simulink model "up_counter_3bit"  (R2025b)
settings: Solver=VariableStepAuto  StartTime=0.0  StopTime=10.0  RelTol=1e-3
libraries: simulink_extras x4
settings Model: Creator=Johan  LastModifiedBy=Johan

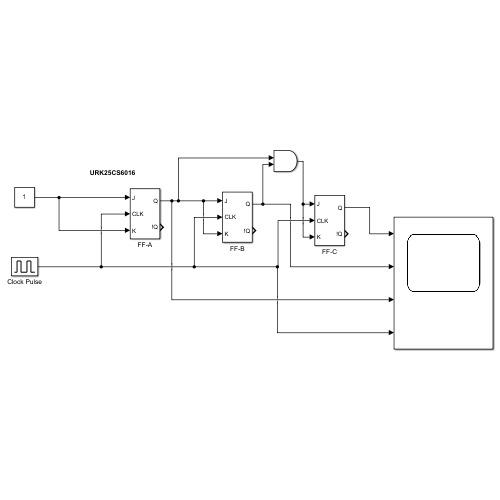
[thumbnail: Simulink's stored preview of the top-level diagram]
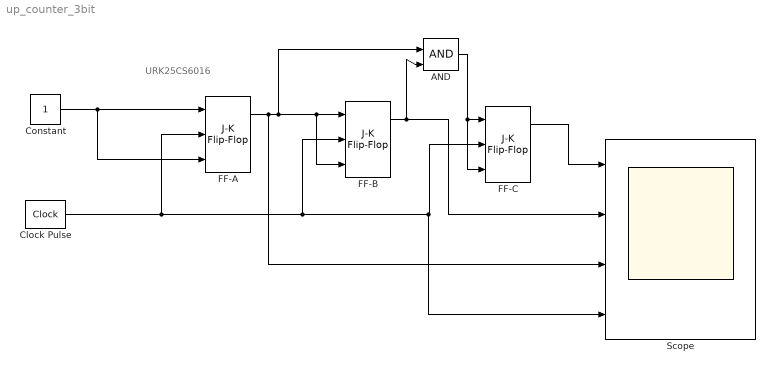
== system up_counter_3bit ==
  note: URK25CS6016
  AND : Logic  IconShape=distinctive  AllPortsSameDT=off  OutDataTypeStr=boolean
  Clock Pulse : simulink_extras/Flip Flops/Clock  period=2
  Constant : Constant  OutDataTypeStr=boolean
  FF-A : simulink_extras/Flip Flops/J-K Flip-Flop  initial_condition=0
  FF-B : simulink_extras/Flip Flops/J-K Flip-Flop  initial_condition=0
  FF-C : simulink_extras/Flip Flops/J-K Flip-Flop  initial_condition=0
  Scope : Scope  NumInputPorts=4
      settings: ActiveDisplayYMinimum=-0.12499999999999997  ActiveDisplayYMaximum=1.125
  wires:
  FF-A/1 -> FF-B/1, FF-B/3, AND/1, Scope/3
  FF-C/1 -> Scope/1
  Constant/1 -> FF-A/3, FF-A/1
  AND/1 -> FF-C/3, FF-C/1
  Clock Pulse/1 -> Scope/4, FF-C/2, FF-B/2, FF-A/2
  FF-B/1 -> Scope/2, AND/2
